simulink model "Demo_CooperativeDriving_cs"  (R2014b)
settings: Solver=ode5  SolverMode=SingleTasking  StartTime=0.0  StopTime=8  FixedStep=1/20  RelTol=1e-3
PreLoadFcn:
  | mbxruntime.callbacks.PreLoadFcn(bdroot);
  | check_NUTS_defined
  | model_closed = 0;
  | assignin('base',['model_closed_' bdroot],false);
PostLoadFcn:
  | mbxruntime.callbacks.PostLoadFcn(bdroot);
InitFcn:
  | mbxruntime.callbacks.InitFcn(bdroot);
StartFcn:
  | mbxruntime.callbacks.StartFcn(bdroot);
StopFcn:
  | mbxruntime.callbacks.StopFcn(bdroot);;
  | 
model workspace: external: MAT-File .\Demo_CooperativeDriving_cs_hws.mat (data not in the file)
undefined symbols (not defined in the file or in its folder): Cf, Cr, Jzz, Kaa, Kf, Kr, Kva, laa, lva, m, Mu, relax_on, sigma_f, sigma_r, TyreType
undefined symbols (not defined in the file): Demo_CooperativeDriving_cs_019e31e1e3c8ec68, Demo_CooperativeDriving_cs_06ab175f8e490aca, Demo_CooperativeDriving_cs_0e8790fd2fe2c963, Demo_CooperativeDriving_cs_18427a499ef3a070, Demo_CooperativeDriving_cs_19ee9ca2bc3a81c5, Demo_CooperativeDriving_cs_1e89904560c1227b, Demo_CooperativeDriving_cs_2a21be70e9dcad5a, Demo_CooperativeDriving_cs_3c5a74ebc1eb48ac, Demo_CooperativeDriving_cs_3ecaa3121594636b, Demo_CooperativeDriving_cs_43d52ce951fced72, Demo_CooperativeDriving_cs_475d8ea73085ad3a, Demo_CooperativeDriving_cs_4c403bcd11f4ac48, Demo_CooperativeDriving_cs_500af6239feadecf, Demo_CooperativeDriving_cs_53c9d62e9dff8a3d, Demo_CooperativeDriving_cs_63d3785fefec7df9, Demo_CooperativeDriving_cs_65798d17832a6887, Demo_CooperativeDriving_cs_684f3b729e0e35ac, Demo_CooperativeDriving_cs_7b7020bcdeec0410, Demo_CooperativeDriving_cs_803ec305ff24ac25, Demo_CooperativeDriving_cs_91ed94aee88cd921, Demo_CooperativeDriving_cs_9556f9105729d50c, Demo_CooperativeDriving_cs_9c65d481a76c7229, Demo_CooperativeDriving_cs_a1df81188d2866f5, Demo_CooperativeDriving_cs_a568973dc598679c, Demo_CooperativeDriving_cs_a8d1daa2431509ff, Demo_CooperativeDriving_cs_b3151f9b5b26be37, Demo_CooperativeDriving_cs_b4ba40b0a5f80027, Demo_CooperativeDriving_cs_c063d1b03f7840be, Demo_CooperativeDriving_cs_d5243d3d2f20e205, Demo_CooperativeDriving_cs_e247c6181801d737, Demo_CooperativeDriving_cs_fb1b7b87fe1ec171, Demo_CooperativeDriving_cs_Mazda_RX8_1_Path_pathUniqueID
libraries: PreScanSimulinkLibrary x10, simulink_extras x5
(part 5 of 5)

== system Demo_CooperativeDriving_cs/Toyota_Previa_1/SELF_Demux/compas converter/cart2compas ==
  Angle [deg] : Inport
  Constant : Constant  Value=90
  Constant1 : Constant  Value=360
  Gain : Gain  Gain=1/360
  Gain1 : Gain  Gain=360
  Gain2 : Gain  Gain=-1
  Rounding Function : Rounding
  Sum : Sum  Inputs=|-+
  Sum1 : Sum  Inputs=-+|
  Sum2 : Sum  Inputs=++|
  heading [deg] : Outport
  wires:
  Gain/1 -> Rounding Function/1
  Rounding Function/1 -> Gain1/1
  Gain1/1 -> Sum/1
  Angle [deg]/1 -> Sum1/2
  Sum/1 -> Gain2/1
  Sum1/1 -> Gain/1, Sum/2
  Constant/1 -> Sum1/1
  Gain2/1 -> Sum2/2
  Constant1/1 -> Sum2/1
  Sum2/1 -> heading [deg]/1

== system Demo_CooperativeDriving_cs/Toyota_Previa_1/Swarm Behavior/Vehicle/eq_of_motion ==
  Vx : Inport
  F_lat : Inport  Port=2
  Mz : Inport  Port=3
  Fcn1 : Fcn  Expr=u(1)*u(3)
  Gain : Gain  Gain=1/m  SaturateOnIntegerOverflow=on  OutDataTypeStr=Inherit: Same as input  ParamDataTypeStr=Inherit: Same as input
  Gain1 : Gain  Gain=1/Jzz  SaturateOnIntegerOverflow=on  OutDataTypeStr=Inherit: Same as input  ParamDataTypeStr=Inherit: Same as input
  Integrator1 : Integrator
  Integrator4 : Integrator
  Integrator5 : Integrator
  Psip : Integrator
  Sum1 : Sum  Inputs=-+  SaturateOnIntegerOverflow=on  InputSameDT=on  OutDataTypeStr=Inherit: Same as first input
  Vx0 : Fcn  Expr=u(1)*cos(u(3)) - u(2)*sin(u(3))
  "Vy " : Integrator
  Vy0 : Fcn  Expr=u(1)*sin(u(3)) + u(2)*cos(u(3))
  X3 : Mux  Inputs=3
  Xp : Mux  Inputs=3
  Xp1 : Mux  Inputs=2
  Xp2 : Mux  Inputs=3
  x_y_psi : Outport  InitialOutput=0
  dx_dy_dpsi : Outport  Port=2  InitialOutput=0
  ddy_ddpsi : Outport  Port=3  InitialOutput=0
  wires:
  Integrator1/1 -> X3/3, Xp2/3  "psi"
  X3/1 -> x_y_psi/1
  Integrator4/1 -> X3/1  "x"
  Integrator5/1 -> X3/2  "y"
  Vy0/1 -> Integrator5/1
  Vx0/1 -> Integrator4/1
  Xp2/1 -> Vy0/1, Vx0/1
  Mz/1 -> Gain1/1
  Xp1/1 -> ddy_ddpsi/1
  F_lat/1 -> Gain/1
  Sum1/1 -> Xp1/1, "Vy "/1  "dd_y"
  Fcn1/1 -> Sum1/1
  Xp/1 -> dx_dy_dpsi/1, Fcn1/1
  Gain1/1 -> Xp1/2, Psip/1  "dd_psi"
  Vx/1 -> Xp2/1, Xp/1
  Gain/1 -> Sum1/2
  "Vy "/1 -> Xp2/2, Xp/2  "d_y"
  Psip/1 -> Integrator1/1, Xp/3  "d_psi"

== system Demo_CooperativeDriving_cs/Toyota_Previa_1/Swarm Behavior/Vehicle/slip_angles ==
  note: relax_on
      | ON: 1
      | OFF: 0
  dx_dy_dpsi : Inport
  delta : Inport  Port=2
  Constant : Constant  Value=relax_on
  Constant1 : Constant  Value=relax_on
  Mux2 : Mux  Inputs=2
  Sum : Sum  Inputs=++|  SaturateOnIntegerOverflow=on  InputSameDT=on  OutDataTypeStr=Inherit: Same as first input
  Switch : Switch  Threshold=0.5  SaturateOnIntegerOverflow=on  InputSameDT=on
  Switch1 : Switch  Threshold=0.5  SaturateOnIntegerOverflow=on  InputSameDT=on
  alpha_front : Fcn  Expr=-atan( (u(2)+u(3)*lva)/u(1) )
  alpha_rear : Fcn  Expr=-atan( (u(2)-u(3)*laa)/u(1) )
  relaxation_length_front : Subsystem
  relaxation_length_rear : Subsystem
  alpha : Outport
  wires:
  Constant/1 -> Switch/2
  Constant1/1 -> Switch1/2
  Switch1/1 -> Mux2/2  "alpha_r"
  Switch/1 -> Mux2/1  "alpha_f"
  relaxation_length_rear/1(alpha_relax) -> Switch1/1
  relaxation_length_front/1(alpha_relax) -> Switch/1
  alpha_rear/1 -> Switch1/3, relaxation_length_rear/1(alpha_stat)  "alpha_stat_r"
  Sum/1 -> Switch/3, relaxation_length_front/1(alpha_stat)  "alpha_stat_f"
  Mux2/1 -> alpha/1
  dx_dy_dpsi/1 -> relaxation_length_rear/2(dx,dy,dphi), alpha_rear/1, relaxation_length_front/2(dx,dy,dphi), alpha_front/1
  delta/1 -> Sum/1
  alpha_front/1 -> Sum/2

== system Demo_CooperativeDriving_cs/Toyota_Previa_1/Swarm Behavior/Vehicle/tyre_forces ==
  alpha : Inport
  delta : Inport  Port=2
  Demux1 : Demux  Outputs=2
  Fy : Fcn  Expr=u(2)*cos(u(1)) + u(3)
  M2 : Fcn  Expr=u(2)*lva*cos(u(1)) - u(3)*laa
  Mux : Mux  Inputs=2
  Mux2 : Mux  Inputs=3
  tyre_front : Subsystem
  tyre_rear : Subsystem
  Fy_wheels : Outport  InitialOutput=0
  F_lat : Outport  Port=2  InitialOutput=0
  Mz : Outport  Port=3  InitialOutput=0
  wires:
  delta/1 -> Mux2/1
  tyre_rear/1(Fy_r) -> Mux/2, Mux2/3  "Fy_r"
  tyre_front/1(Fy_f) -> Mux/1, Mux2/2  "Fy_f"
  Demux1/2 -> tyre_rear/1(alpha)
  Demux1/1 -> tyre_front/1(alpha)
  alpha/1 -> Demux1/1
  Mux2/1 -> Fy/1, M2/1
  Fy/1 -> F_lat/1
  M2/1 -> Mz/1
  Mux/1 -> Fy_wheels/1

== system Demo_CooperativeDriving_cs/Toyota_Yaris_1/SELF_Demux/compas converter/cart2compas ==
  Angle [deg] : Inport
  Constant : Constant  Value=90
  Constant1 : Constant  Value=360
  Gain : Gain  Gain=1/360
  Gain1 : Gain  Gain=360
  Gain2 : Gain  Gain=-1
  Rounding Function : Rounding
  Sum : Sum  Inputs=|-+
  Sum1 : Sum  Inputs=-+|
  Sum2 : Sum  Inputs=++|
  heading [deg] : Outport
  wires:
  Gain/1 -> Rounding Function/1
  Rounding Function/1 -> Gain1/1
  Gain1/1 -> Sum/1
  Angle [deg]/1 -> Sum1/2
  Sum/1 -> Gain2/1
  Sum1/1 -> Gain/1, Sum/2
  Constant/1 -> Sum1/1
  Gain2/1 -> Sum2/2
  Constant1/1 -> Sum2/1
  Sum2/1 -> heading [deg]/1

== system Demo_CooperativeDriving_cs/Toyota_Yaris_1/Swarm Behavior/Vehicle Dynamics/eq_of_motion ==
  Vx : Inport
  F_lat : Inport  Port=2
  Mz : Inport  Port=3
  Fcn1 : Fcn  Expr=u(1)*u(3)
  Gain : Gain  Gain=1/m  SaturateOnIntegerOverflow=on  OutDataTypeStr=Inherit: Same as input  ParamDataTypeStr=Inherit: Same as input
  Gain1 : Gain  Gain=1/Jzz  SaturateOnIntegerOverflow=on  OutDataTypeStr=Inherit: Same as input  ParamDataTypeStr=Inherit: Same as input
  Integrator1 : Integrator
  Integrator4 : Integrator
  Integrator5 : Integrator
  Psip : Integrator
  Sum1 : Sum  Inputs=-+  SaturateOnIntegerOverflow=on  InputSameDT=on  OutDataTypeStr=Inherit: Same as first input
  Vx0 : Fcn  Expr=u(1)*cos(u(3)) - u(2)*sin(u(3))
  "Vy " : Integrator
  Vy0 : Fcn  Expr=u(1)*sin(u(3)) + u(2)*cos(u(3))
  X3 : Mux  Inputs=3
  Xp : Mux  Inputs=3
  Xp1 : Mux  Inputs=2
  Xp2 : Mux  Inputs=3
  x_y_psi : Outport  InitialOutput=0
  dx_dy_dpsi : Outport  Port=2  InitialOutput=0
  ddy_ddpsi : Outport  Port=3  InitialOutput=0
  wires:
  Integrator1/1 -> X3/3, Xp2/3  "psi"
  X3/1 -> x_y_psi/1
  Integrator4/1 -> X3/1  "x"
  Integrator5/1 -> X3/2  "y"
  Vy0/1 -> Integrator5/1
  Vx0/1 -> Integrator4/1
  Xp2/1 -> Vy0/1, Vx0/1
  Mz/1 -> Gain1/1
  Xp1/1 -> ddy_ddpsi/1
  F_lat/1 -> Gain/1
  Sum1/1 -> Xp1/1, "Vy "/1  "dd_y"
  Fcn1/1 -> Sum1/1
  Xp/1 -> dx_dy_dpsi/1, Fcn1/1
  Gain1/1 -> Xp1/2, Psip/1  "dd_psi"
  Vx/1 -> Xp2/1, Xp/1
  Gain/1 -> Sum1/2
  "Vy "/1 -> Xp2/2, Xp/2  "d_y"
  Psip/1 -> Integrator1/1, Xp/3  "d_psi"

== system Demo_CooperativeDriving_cs/Toyota_Yaris_1/Swarm Behavior/Vehicle Dynamics/slip_angles ==
  note: relax_on
      | ON: 1
      | OFF: 0
  dx_dy_dpsi : Inport
  delta : Inport  Port=2
  Constant : Constant  Value=relax_on
  Constant1 : Constant  Value=relax_on
  Mux2 : Mux  Inputs=2
  Sum : Sum  Inputs=++|  SaturateOnIntegerOverflow=on  InputSameDT=on  OutDataTypeStr=Inherit: Same as first input
  Switch : Switch  Threshold=0.5  SaturateOnIntegerOverflow=on  InputSameDT=on
  Switch1 : Switch  Threshold=0.5  SaturateOnIntegerOverflow=on  InputSameDT=on
  alpha_front : Fcn  Expr=-atan( (u(2)+u(3)*lva)/u(1) )
  alpha_rear : Fcn  Expr=-atan( (u(2)-u(3)*laa)/u(1) )
  relaxation_length_front : Subsystem
  relaxation_length_rear : Subsystem
  alpha : Outport
  wires:
  Constant/1 -> Switch/2
  Constant1/1 -> Switch1/2
  Switch1/1 -> Mux2/2  "alpha_r"
  Switch/1 -> Mux2/1  "alpha_f"
  relaxation_length_rear/1(alpha_relax) -> Switch1/1
  relaxation_length_front/1(alpha_relax) -> Switch/1
  alpha_rear/1 -> Switch1/3, relaxation_length_rear/1(alpha_stat)  "alpha_stat_r"
  Sum/1 -> Switch/3, relaxation_length_front/1(alpha_stat)  "alpha_stat_f"
  Mux2/1 -> alpha/1
  dx_dy_dpsi/1 -> relaxation_length_rear/2(dx,dy,dphi), alpha_rear/1, relaxation_length_front/2(dx,dy,dphi), alpha_front/1
  delta/1 -> Sum/1
  alpha_front/1 -> Sum/2

== system Demo_CooperativeDriving_cs/Toyota_Yaris_1/Swarm Behavior/Vehicle Dynamics/tyre_forces ==
  alpha : Inport
  delta : Inport  Port=2
  Demux1 : Demux  Outputs=2
  Fy : Fcn  Expr=u(2)*cos(u(1)) + u(3)
  M2 : Fcn  Expr=u(2)*lva*cos(u(1)) - u(3)*laa
  Mux : Mux  Inputs=2
  Mux2 : Mux  Inputs=3
  tyre_front : Subsystem
  tyre_rear : Subsystem
  Fy_wheels : Outport  InitialOutput=0
  F_lat : Outport  Port=2  InitialOutput=0
  Mz : Outport  Port=3  InitialOutput=0
  wires:
  delta/1 -> Mux2/1
  tyre_rear/1(Fy_r) -> Mux/2, Mux2/3  "Fy_r"
  tyre_front/1(Fy_f) -> Mux/1, Mux2/2  "Fy_f"
  Demux1/2 -> tyre_rear/1(alpha)
  Demux1/1 -> tyre_front/1(alpha)
  alpha/1 -> Demux1/1
  Mux2/1 -> Fy/1, M2/1
  Fy/1 -> F_lat/1
  M2/1 -> Mz/1
  Mux/1 -> Fy_wheels/1

== system Demo_CooperativeDriving_cs/BMW_X5_1/Swarm Behavior/Vehicle Dynamics/slip_angles/relaxation_length_front ==
  alpha_stat : Inport
  dx,dy,dphi : Inport  Port=2
  Integrator : Integrator
  Linl : Fcn  Expr=(u(4) - u(5))/(sigma_f/u(1))
  Mux2 : Mux  Inputs={3,1,1}
  alpha_relax : Outport
  wires:
  alpha_stat/1 -> Mux2/2
  dx,dy,dphi/1 -> Mux2/1
  Integrator/1 -> Mux2/3, alpha_relax/1
  Linl/1 -> Integrator/1
  Mux2/1 -> Linl/1

== system Demo_CooperativeDriving_cs/BMW_X5_1/Swarm Behavior/Vehicle Dynamics/slip_angles/relaxation_length_rear ==
  alpha_stat : Inport
  dx,dy,dphi : Inport  Port=2
  Integrator : Integrator
  Linl : Fcn  Expr=(u(4) - u(5))/(sigma_r/u(1))
  Mux2 : Mux  Inputs={3,1,1}
  alpha_relax : Outport
  wires:
  alpha_stat/1 -> Mux2/2
  dx,dy,dphi/1 -> Mux2/1
  Integrator/1 -> Mux2/3, alpha_relax/1
  Linl/1 -> Integrator/1
  Mux2/1 -> Linl/1

== system Demo_CooperativeDriving_cs/BMW_X5_1/Swarm Behavior/Vehicle Dynamics/tyre_forces/tyre_front ==
  alpha : Inport
  Borstel : Subsystem
  Exponent : Subsystem
  Fva : Fcn  Expr=Kva*u
  Fz : Constant  Value=2*Cf
  Kf : Constant  Value=Kf
  Mu : Constant  Value=Mu
  Multiport Switch : MultiPortSwitch  SaturateOnIntegerOverflow=on  InputSameDT=on
  Type : Constant  Value=TyreType
  Fy_f : Outport  InitialOutput=0
  wires:
  Fz/1 -> Exponent/2(Fz), Borstel/2(Fz)
  Mu/1 -> Exponent/3(Mu), Borstel/3(Mu)
  alpha/1 -> Fva/1, Exponent/1(alpha), Borstel/1(alpha)
  Kf/1 -> Exponent/4(Kt), Borstel/4(Kt)
  Borstel/1(Fy) -> Multiport Switch/4
  Exponent/1(Fy) -> Multiport Switch/3
  Fva/1 -> Multiport Switch/2
  Multiport Switch/1 -> Fy_f/1
  Type/1 -> Multiport Switch/1

== system Demo_CooperativeDriving_cs/BMW_X5_1/Swarm Behavior/Vehicle Dynamics/tyre_forces/tyre_rear ==
  alpha : Inport
  Borstel : Subsystem
  Exponent : Subsystem
  Fva : Fcn  Expr=Kaa*u
  Fz : Constant  Value=2*Cr
  Kr : Constant  Value=Kr
  Mu : Constant  Value=Mu
  Multiport Switch : MultiPortSwitch  SaturateOnIntegerOverflow=on  InputSameDT=on
  Type : Constant  Value=TyreType
  Fy_r : Outport  InitialOutput=0
  wires:
  alpha/1 -> Fva/1, Exponent/1(alpha), Borstel/1(alpha)
  Fz/1 -> Exponent/2(Fz), Borstel/2(Fz)
  Mu/1 -> Exponent/3(Mu), Borstel/3(Mu)
  Kr/1 -> Exponent/4(Kt), Borstel/4(Kt)
  Borstel/1(Fy) -> Multiport Switch/4
  Exponent/1(Fy) -> Multiport Switch/3
  Fva/1 -> Multiport Switch/2
  Type/1 -> Multiport Switch/1
  Multiport Switch/1 -> Fy_r/1

== system Demo_CooperativeDriving_cs/Citroen_C3_1/Swarm Behavior/Vehicle Dynamics/slip_angles/relaxation_length_front ==
  alpha_stat : Inport
  dx,dy,dphi : Inport  Port=2
  Integrator : Integrator
  Linl : Fcn  Expr=(u(4) - u(5))/(sigma_f/u(1))
  Mux2 : Mux  Inputs={3,1,1}
  alpha_relax : Outport
  wires:
  alpha_stat/1 -> Mux2/2
  dx,dy,dphi/1 -> Mux2/1
  Integrator/1 -> Mux2/3, alpha_relax/1
  Linl/1 -> Integrator/1
  Mux2/1 -> Linl/1

== system Demo_CooperativeDriving_cs/Citroen_C3_1/Swarm Behavior/Vehicle Dynamics/slip_angles/relaxation_length_rear ==
  alpha_stat : Inport
  dx,dy,dphi : Inport  Port=2
  Integrator : Integrator
  Linl : Fcn  Expr=(u(4) - u(5))/(sigma_r/u(1))
  Mux2 : Mux  Inputs={3,1,1}
  alpha_relax : Outport
  wires:
  alpha_stat/1 -> Mux2/2
  dx,dy,dphi/1 -> Mux2/1
  Integrator/1 -> Mux2/3, alpha_relax/1
  Linl/1 -> Integrator/1
  Mux2/1 -> Linl/1

== system Demo_CooperativeDriving_cs/Citroen_C3_1/Swarm Behavior/Vehicle Dynamics/tyre_forces/tyre_front ==
  alpha : Inport
  Borstel : Subsystem
  Exponent : Subsystem
  Fva : Fcn  Expr=Kva*u
  Fz : Constant  Value=2*Cf
  Kf : Constant  Value=Kf
  Mu : Constant  Value=Mu
  Multiport Switch : MultiPortSwitch  SaturateOnIntegerOverflow=on  InputSameDT=on
  Type : Constant  Value=TyreType
  Fy_f : Outport  InitialOutput=0
  wires:
  Fz/1 -> Exponent/2(Fz), Borstel/2(Fz)
  Mu/1 -> Exponent/3(Mu), Borstel/3(Mu)
  alpha/1 -> Fva/1, Exponent/1(alpha), Borstel/1(alpha)
  Kf/1 -> Exponent/4(Kt), Borstel/4(Kt)
  Borstel/1(Fy) -> Multiport Switch/4
  Exponent/1(Fy) -> Multiport Switch/3
  Fva/1 -> Multiport Switch/2
  Multiport Switch/1 -> Fy_f/1
  Type/1 -> Multiport Switch/1

== system Demo_CooperativeDriving_cs/Citroen_C3_1/Swarm Behavior/Vehicle Dynamics/tyre_forces/tyre_rear ==
  alpha : Inport
  Borstel : Subsystem
  Exponent : Subsystem
  Fva : Fcn  Expr=Kaa*u
  Fz : Constant  Value=2*Cr
  Kr : Constant  Value=Kr
  Mu : Constant  Value=Mu
  Multiport Switch : MultiPortSwitch  SaturateOnIntegerOverflow=on  InputSameDT=on
  Type : Constant  Value=TyreType
  Fy_r : Outport  InitialOutput=0
  wires:
  alpha/1 -> Fva/1, Exponent/1(alpha), Borstel/1(alpha)
  Fz/1 -> Exponent/2(Fz), Borstel/2(Fz)
  Mu/1 -> Exponent/3(Mu), Borstel/3(Mu)
  Kr/1 -> Exponent/4(Kt), Borstel/4(Kt)
  Borstel/1(Fy) -> Multiport Switch/4
  Exponent/1(Fy) -> Multiport Switch/3
  Fva/1 -> Multiport Switch/2
  Type/1 -> Multiport Switch/1
  Multiport Switch/1 -> Fy_r/1

== system Demo_CooperativeDriving_cs/Nissan_Cabstar_1/Swarm Behavior/Vehicle Dynamics/slip_angles/relaxation_length_front ==
  alpha_stat : Inport
  dx,dy,dphi : Inport  Port=2
  Integrator : Integrator
  Linl : Fcn  Expr=(u(4) - u(5))/(sigma_f/u(1))
  Mux2 : Mux  Inputs={3,1,1}
  alpha_relax : Outport
  wires:
  alpha_stat/1 -> Mux2/2
  dx,dy,dphi/1 -> Mux2/1
  Integrator/1 -> Mux2/3, alpha_relax/1
  Linl/1 -> Integrator/1
  Mux2/1 -> Linl/1

== system Demo_CooperativeDriving_cs/Nissan_Cabstar_1/Swarm Behavior/Vehicle Dynamics/slip_angles/relaxation_length_rear ==
  alpha_stat : Inport
  dx,dy,dphi : Inport  Port=2
  Integrator : Integrator
  Linl : Fcn  Expr=(u(4) - u(5))/(sigma_r/u(1))
  Mux2 : Mux  Inputs={3,1,1}
  alpha_relax : Outport
  wires:
  alpha_stat/1 -> Mux2/2
  dx,dy,dphi/1 -> Mux2/1
  Integrator/1 -> Mux2/3, alpha_relax/1
  Linl/1 -> Integrator/1
  Mux2/1 -> Linl/1

== system Demo_CooperativeDriving_cs/Nissan_Cabstar_1/Swarm Behavior/Vehicle Dynamics/tyre_forces/tyre_front ==
  alpha : Inport
  Borstel : Subsystem
  Exponent : Subsystem
  Fva : Fcn  Expr=Kva*u
  Fz : Constant  Value=2*Cf
  Kf : Constant  Value=Kf
  Mu : Constant  Value=Mu
  Multiport Switch : MultiPortSwitch  SaturateOnIntegerOverflow=on  InputSameDT=on
  Type : Constant  Value=TyreType
  Fy_f : Outport  InitialOutput=0
  wires:
  Fz/1 -> Exponent/2(Fz), Borstel/2(Fz)
  Mu/1 -> Exponent/3(Mu), Borstel/3(Mu)
  alpha/1 -> Fva/1, Exponent/1(alpha), Borstel/1(alpha)
  Kf/1 -> Exponent/4(Kt), Borstel/4(Kt)
  Borstel/1(Fy) -> Multiport Switch/4
  Exponent/1(Fy) -> Multiport Switch/3
  Fva/1 -> Multiport Switch/2
  Multiport Switch/1 -> Fy_f/1
  Type/1 -> Multiport Switch/1

== system Demo_CooperativeDriving_cs/Nissan_Cabstar_1/Swarm Behavior/Vehicle Dynamics/tyre_forces/tyre_rear ==
  alpha : Inport
  Borstel : Subsystem
  Exponent : Subsystem
  Fva : Fcn  Expr=Kaa*u
  Fz : Constant  Value=2*Cr
  Kr : Constant  Value=Kr
  Mu : Constant  Value=Mu
  Multiport Switch : MultiPortSwitch  SaturateOnIntegerOverflow=on  InputSameDT=on
  Type : Constant  Value=TyreType
  Fy_r : Outport  InitialOutput=0
  wires:
  alpha/1 -> Fva/1, Exponent/1(alpha), Borstel/1(alpha)
  Fz/1 -> Exponent/2(Fz), Borstel/2(Fz)
  Mu/1 -> Exponent/3(Mu), Borstel/3(Mu)
  Kr/1 -> Exponent/4(Kt), Borstel/4(Kt)
  Borstel/1(Fy) -> Multiport Switch/4
  Exponent/1(Fy) -> Multiport Switch/3
  Fva/1 -> Multiport Switch/2
  Type/1 -> Multiport Switch/1
  Multiport Switch/1 -> Fy_r/1

== system Demo_CooperativeDriving_cs/Toyota_Previa_1/Swarm Behavior/Vehicle/slip_angles/relaxation_length_front ==
  alpha_stat : Inport
  dx,dy,dphi : Inport  Port=2
  Integrator : Integrator
  Linl : Fcn  Expr=(u(4) - u(5))/(sigma_f/u(1))
  Mux2 : Mux  Inputs={3,1,1}
  alpha_relax : Outport
  wires:
  alpha_stat/1 -> Mux2/2
  dx,dy,dphi/1 -> Mux2/1
  Integrator/1 -> Mux2/3, alpha_relax/1
  Linl/1 -> Integrator/1
  Mux2/1 -> Linl/1

== system Demo_CooperativeDriving_cs/Toyota_Previa_1/Swarm Behavior/Vehicle/slip_angles/relaxation_length_rear ==
  alpha_stat : Inport
  dx,dy,dphi : Inport  Port=2
  Integrator : Integrator
  Linl : Fcn  Expr=(u(4) - u(5))/(sigma_r/u(1))
  Mux2 : Mux  Inputs={3,1,1}
  alpha_relax : Outport
  wires:
  alpha_stat/1 -> Mux2/2
  dx,dy,dphi/1 -> Mux2/1
  Integrator/1 -> Mux2/3, alpha_relax/1
  Linl/1 -> Integrator/1
  Mux2/1 -> Linl/1

== system Demo_CooperativeDriving_cs/Toyota_Previa_1/Swarm Behavior/Vehicle/tyre_forces/tyre_front ==
  alpha : Inport
  Borstel : Subsystem
  Exponent : Subsystem
  Fva : Fcn  Expr=Kva*u
  Fz : Constant  Value=2*Cf
  Kf : Constant  Value=Kf
  Mu : Constant  Value=Mu
  Multiport Switch : MultiPortSwitch  SaturateOnIntegerOverflow=on  InputSameDT=on
  Type : Constant  Value=TyreType
  Fy_f : Outport  InitialOutput=0
  wires:
  Fz/1 -> Exponent/2(Fz), Borstel/2(Fz)
  Mu/1 -> Exponent/3(Mu), Borstel/3(Mu)
  alpha/1 -> Fva/1, Exponent/1(alpha), Borstel/1(alpha)
  Kf/1 -> Exponent/4(Kt), Borstel/4(Kt)
  Borstel/1(Fy) -> Multiport Switch/4
  Exponent/1(Fy) -> Multiport Switch/3
  Fva/1 -> Multiport Switch/2
  Multiport Switch/1 -> Fy_f/1
  Type/1 -> Multiport Switch/1

== system Demo_CooperativeDriving_cs/Toyota_Previa_1/Swarm Behavior/Vehicle/tyre_forces/tyre_rear ==
  alpha : Inport
  Borstel : Subsystem
  Exponent : Subsystem
  Fva : Fcn  Expr=Kaa*u
  Fz : Constant  Value=2*Cr
  Kr : Constant  Value=Kr
  Mu : Constant  Value=Mu
  Multiport Switch : MultiPortSwitch  SaturateOnIntegerOverflow=on  InputSameDT=on
  Type : Constant  Value=TyreType
  Fy_r : Outport  InitialOutput=0
  wires:
  alpha/1 -> Fva/1, Exponent/1(alpha), Borstel/1(alpha)
  Fz/1 -> Exponent/2(Fz), Borstel/2(Fz)
  Mu/1 -> Exponent/3(Mu), Borstel/3(Mu)
  Kr/1 -> Exponent/4(Kt), Borstel/4(Kt)
  Borstel/1(Fy) -> Multiport Switch/4
  Exponent/1(Fy) -> Multiport Switch/3
  Fva/1 -> Multiport Switch/2
  Type/1 -> Multiport Switch/1
  Multiport Switch/1 -> Fy_r/1

== system Demo_CooperativeDriving_cs/Toyota_Yaris_1/Swarm Behavior/Vehicle Dynamics/slip_angles/relaxation_length_front ==
  alpha_stat : Inport
  dx,dy,dphi : Inport  Port=2
  Integrator : Integrator
  Linl : Fcn  Expr=(u(4) - u(5))/(sigma_f/u(1))
  Mux2 : Mux  Inputs={3,1,1}
  alpha_relax : Outport
  wires:
  alpha_stat/1 -> Mux2/2
  dx,dy,dphi/1 -> Mux2/1
  Integrator/1 -> Mux2/3, alpha_relax/1
  Linl/1 -> Integrator/1
  Mux2/1 -> Linl/1

== system Demo_CooperativeDriving_cs/Toyota_Yaris_1/Swarm Behavior/Vehicle Dynamics/slip_angles/relaxation_length_rear ==
  alpha_stat : Inport
  dx,dy,dphi : Inport  Port=2
  Integrator : Integrator
  Linl : Fcn  Expr=(u(4) - u(5))/(sigma_r/u(1))
  Mux2 : Mux  Inputs={3,1,1}
  alpha_relax : Outport
  wires:
  alpha_stat/1 -> Mux2/2
  dx,dy,dphi/1 -> Mux2/1
  Integrator/1 -> Mux2/3, alpha_relax/1
  Linl/1 -> Integrator/1
  Mux2/1 -> Linl/1

== system Demo_CooperativeDriving_cs/Toyota_Yaris_1/Swarm Behavior/Vehicle Dynamics/tyre_forces/tyre_front ==
  alpha : Inport
  Borstel : Subsystem
  Exponent : Subsystem
  Fva : Fcn  Expr=Kva*u
  Fz : Constant  Value=2*Cf
  Kf : Constant  Value=Kf
  Mu : Constant  Value=Mu
  Multiport Switch : MultiPortSwitch  SaturateOnIntegerOverflow=on  InputSameDT=on
  Type : Constant  Value=TyreType
  Fy_f : Outport  InitialOutput=0
  wires:
  Fz/1 -> Exponent/2(Fz), Borstel/2(Fz)
  Mu/1 -> Exponent/3(Mu), Borstel/3(Mu)
  alpha/1 -> Fva/1, Exponent/1(alpha), Borstel/1(alpha)
  Kf/1 -> Exponent/4(Kt), Borstel/4(Kt)
  Borstel/1(Fy) -> Multiport Switch/4
  Exponent/1(Fy) -> Multiport Switch/3
  Fva/1 -> Multiport Switch/2
  Multiport Switch/1 -> Fy_f/1
  Type/1 -> Multiport Switch/1

== system Demo_CooperativeDriving_cs/Toyota_Yaris_1/Swarm Behavior/Vehicle Dynamics/tyre_forces/tyre_rear ==
  alpha : Inport
  Borstel : Subsystem
  Exponent : Subsystem
  Fva : Fcn  Expr=Kaa*u
  Fz : Constant  Value=2*Cr
  Kr : Constant  Value=Kr
  Mu : Constant  Value=Mu
  Multiport Switch : MultiPortSwitch  SaturateOnIntegerOverflow=on  InputSameDT=on
  Type : Constant  Value=TyreType
  Fy_r : Outport  InitialOutput=0
  wires:
  alpha/1 -> Fva/1, Exponent/1(alpha), Borstel/1(alpha)
  Fz/1 -> Exponent/2(Fz), Borstel/2(Fz)
  Mu/1 -> Exponent/3(Mu), Borstel/3(Mu)
  Kr/1 -> Exponent/4(Kt), Borstel/4(Kt)
  Borstel/1(Fy) -> Multiport Switch/4
  Exponent/1(Fy) -> Multiport Switch/3
  Fva/1 -> Multiport Switch/2
  Type/1 -> Multiport Switch/1
  Multiport Switch/1 -> Fy_r/1

== system Demo_CooperativeDriving_cs/BMW_X5_1/Swarm Behavior/Vehicle Dynamics/tyre_forces/tyre_front/Borstel ==
  alpha : Inport
  Fz : Inport  Port=2
  Mu : Inport  Port=3
  Kt : Inport  Port=4
  Abs : Abs  SaturateOnIntegerOverflow=on
  F : Fcn  Expr=(3*u(2) - 3*u(2)^2 + u(2)^3)*u(1)
  Fmax : Fcn  Expr=u(1)
  Gain : Gain  Gain=1/3  SaturateOnIntegerOverflow=on  OutDataTypeStr=Inherit: Same as input  ParamDataTypeStr=Inherit: Same as input
  Math Function : Math  Operator=reciprocal  SaturateOnIntegerOverflow=on
  Mux1 : Mux  Inputs=2
  Product : Product  SaturateOnIntegerOverflow=on  RndMeth=Zero  InputSameDT=on  OutDataTypeStr=Inherit: Same as first input
  Product1 : Product  Inputs=3  SaturateOnIntegerOverflow=on  RndMeth=Zero  InputSameDT=on  OutDataTypeStr=Inherit: Same as first input
  Relational Operator : RelationalOperator  InputSameDT=on
  Sign : Signum
  Switch : Switch  Threshold=0.5  SaturateOnIntegerOverflow=on  InputSameDT=on
  Trigonometric Function : Trigonometry  Operator=tan
  Fy : Outport
  wires:
  Abs/1 -> Relational Operator/1, Product/1
  Kt/1 -> Gain/1
  Relational Operator/1 -> Switch/2
  Trigonometric Function/1 -> Abs/1
  Mux1/1 -> F/1, Fmax/1
  Sign/1 -> Mux1/1
  Product/1 -> Mux1/2
  F/1 -> Switch/3
  Fmax/1 -> Switch/1
  alpha/1 -> Trigonometric Function/1, Sign/1
  Switch/1 -> Product1/1
  Product1/1 -> Fy/1
  Fz/1 -> Product1/2
  Mu/1 -> Product1/3
  Gain/1 -> Product/2, Math Function/1
  Math Function/1 -> Relational Operator/2

== system Demo_CooperativeDriving_cs/BMW_X5_1/Swarm Behavior/Vehicle Dynamics/tyre_forces/tyre_front/Exponent ==
  alpha : Inport
  Fz : Inport  Port=2
  Mu : Inport  Port=3
  Kt : Inport  Port=4
  Abs : Abs  SaturateOnIntegerOverflow=on
  MuY Front Wheels : Fcn  Expr=(1 - exp(-u(2)*u(1)))
  Mux1 : Mux  Inputs=2
  Product : Product  Inputs=4  SaturateOnIntegerOverflow=on  RndMeth=Zero  InputSameDT=on  OutDataTypeStr=Inherit: Same as first input
  Saturation2 : Saturate  UpperLimit=inf  LowerLimit=1e-9
  Sign : Signum
  Fy : Outport
  wires:
  Abs/1 -> Saturation2/1
  Saturation2/1 -> Mux1/1
  Mux1/1 -> MuY Front Wheels/1
  Kt/1 -> Mux1/2
  Sign/1 -> Product/1
  MuY Front Wheels/1 -> Product/2
  alpha/1 -> Abs/1, Sign/1
  Product/1 -> Fy/1
  Fz/1 -> Product/3
  Mu/1 -> Product/4

== system Demo_CooperativeDriving_cs/BMW_X5_1/Swarm Behavior/Vehicle Dynamics/tyre_forces/tyre_rear/Borstel ==
  alpha : Inport
  Fz : Inport  Port=2
  Mu : Inport  Port=3
  Kt : Inport  Port=4
  Abs : Abs  SaturateOnIntegerOverflow=on
  F : Fcn  Expr=(3*u(2) - 3*u(2)^2 + u(2)^3)*u(1)
  Fmax : Fcn  Expr=u(1)
  Gain : Gain  Gain=1/3  SaturateOnIntegerOverflow=on  OutDataTypeStr=Inherit: Same as input  ParamDataTypeStr=Inherit: Same as input
  Math Function : Math  Operator=reciprocal  SaturateOnIntegerOverflow=on
  Mux1 : Mux  Inputs=2
  Product : Product  SaturateOnIntegerOverflow=on  RndMeth=Zero  InputSameDT=on  OutDataTypeStr=Inherit: Same as first input
  Product1 : Product  Inputs=3  SaturateOnIntegerOverflow=on  RndMeth=Zero  InputSameDT=on  OutDataTypeStr=Inherit: Same as first input
  Relational Operator : RelationalOperator  InputSameDT=on
  Sign : Signum
  Switch : Switch  Threshold=0.5  SaturateOnIntegerOverflow=on  InputSameDT=on
  Trigonometric Function : Trigonometry  Operator=tan
  Fy : Outport
  wires:
  Abs/1 -> Relational Operator/1, Product/1
  Kt/1 -> Gain/1
  Relational Operator/1 -> Switch/2
  Trigonometric Function/1 -> Abs/1
  Mux1/1 -> F/1, Fmax/1
  Sign/1 -> Mux1/1
  Product/1 -> Mux1/2
  F/1 -> Switch/3
  Fmax/1 -> Switch/1
  alpha/1 -> Trigonometric Function/1, Sign/1
  Switch/1 -> Product1/1
  Product1/1 -> Fy/1
  Fz/1 -> Product1/2
  Mu/1 -> Product1/3
  Gain/1 -> Product/2, Math Function/1
  Math Function/1 -> Relational Operator/2

== system Demo_CooperativeDriving_cs/BMW_X5_1/Swarm Behavior/Vehicle Dynamics/tyre_forces/tyre_rear/Exponent ==
  alpha : Inport
  Fz : Inport  Port=2
  Mu : Inport  Port=3
  Kt : Inport  Port=4
  Abs : Abs  SaturateOnIntegerOverflow=on
  MuY Front Wheels : Fcn  Expr=(1 - exp(-u(2)*u(1)))
  Mux1 : Mux  Inputs=2
  Product : Product  Inputs=4  SaturateOnIntegerOverflow=on  RndMeth=Zero  InputSameDT=on  OutDataTypeStr=Inherit: Same as first input
  Saturation2 : Saturate  UpperLimit=inf  LowerLimit=1e-9
  Sign : Signum
  Fy : Outport
  wires:
  Abs/1 -> Saturation2/1
  Saturation2/1 -> Mux1/1
  Mux1/1 -> MuY Front Wheels/1
  Kt/1 -> Mux1/2
  Sign/1 -> Product/1
  MuY Front Wheels/1 -> Product/2
  alpha/1 -> Abs/1, Sign/1
  Product/1 -> Fy/1
  Fz/1 -> Product/3
  Mu/1 -> Product/4

== system Demo_CooperativeDriving_cs/Citroen_C3_1/Swarm Behavior/Vehicle Dynamics/tyre_forces/tyre_front/Borstel ==
  alpha : Inport
  Fz : Inport  Port=2
  Mu : Inport  Port=3
  Kt : Inport  Port=4
  Abs : Abs  SaturateOnIntegerOverflow=on
  F : Fcn  Expr=(3*u(2) - 3*u(2)^2 + u(2)^3)*u(1)
  Fmax : Fcn  Expr=u(1)
  Gain : Gain  Gain=1/3  SaturateOnIntegerOverflow=on  OutDataTypeStr=Inherit: Same as input  ParamDataTypeStr=Inherit: Same as input
  Math Function : Math  Operator=reciprocal  SaturateOnIntegerOverflow=on
  Mux1 : Mux  Inputs=2
  Product : Product  SaturateOnIntegerOverflow=on  RndMeth=Zero  InputSameDT=on  OutDataTypeStr=Inherit: Same as first input
  Product1 : Product  Inputs=3  SaturateOnIntegerOverflow=on  RndMeth=Zero  InputSameDT=on  OutDataTypeStr=Inherit: Same as first input
  Relational Operator : RelationalOperator  InputSameDT=on
  Sign : Signum
  Switch : Switch  Threshold=0.5  SaturateOnIntegerOverflow=on  InputSameDT=on
  Trigonometric Function : Trigonometry  Operator=tan
  Fy : Outport
  wires:
  Abs/1 -> Relational Operator/1, Product/1
  Kt/1 -> Gain/1
  Relational Operator/1 -> Switch/2
  Trigonometric Function/1 -> Abs/1
  Mux1/1 -> F/1, Fmax/1
  Sign/1 -> Mux1/1
  Product/1 -> Mux1/2
  F/1 -> Switch/3
  Fmax/1 -> Switch/1
  alpha/1 -> Trigonometric Function/1, Sign/1
  Switch/1 -> Product1/1
  Product1/1 -> Fy/1
  Fz/1 -> Product1/2
  Mu/1 -> Product1/3
  Gain/1 -> Product/2, Math Function/1
  Math Function/1 -> Relational Operator/2

== system Demo_CooperativeDriving_cs/Citroen_C3_1/Swarm Behavior/Vehicle Dynamics/tyre_forces/tyre_front/Exponent ==
  alpha : Inport
  Fz : Inport  Port=2
  Mu : Inport  Port=3
  Kt : Inport  Port=4
  Abs : Abs  SaturateOnIntegerOverflow=on
  MuY Front Wheels : Fcn  Expr=(1 - exp(-u(2)*u(1)))
  Mux1 : Mux  Inputs=2
  Product : Product  Inputs=4  SaturateOnIntegerOverflow=on  RndMeth=Zero  InputSameDT=on  OutDataTypeStr=Inherit: Same as first input
  Saturation2 : Saturate  UpperLimit=inf  LowerLimit=1e-9
  Sign : Signum
  Fy : Outport
  wires:
  Abs/1 -> Saturation2/1
  Saturation2/1 -> Mux1/1
  Mux1/1 -> MuY Front Wheels/1
  Kt/1 -> Mux1/2
  Sign/1 -> Product/1
  MuY Front Wheels/1 -> Product/2
  alpha/1 -> Abs/1, Sign/1
  Product/1 -> Fy/1
  Fz/1 -> Product/3
  Mu/1 -> Product/4

== system Demo_CooperativeDriving_cs/Citroen_C3_1/Swarm Behavior/Vehicle Dynamics/tyre_forces/tyre_rear/Borstel ==
  alpha : Inport
  Fz : Inport  Port=2
  Mu : Inport  Port=3
  Kt : Inport  Port=4
  Abs : Abs  SaturateOnIntegerOverflow=on
  F : Fcn  Expr=(3*u(2) - 3*u(2)^2 + u(2)^3)*u(1)
  Fmax : Fcn  Expr=u(1)
  Gain : Gain  Gain=1/3  SaturateOnIntegerOverflow=on  OutDataTypeStr=Inherit: Same as input  ParamDataTypeStr=Inherit: Same as input
  Math Function : Math  Operator=reciprocal  SaturateOnIntegerOverflow=on
  Mux1 : Mux  Inputs=2
  Product : Product  SaturateOnIntegerOverflow=on  RndMeth=Zero  InputSameDT=on  OutDataTypeStr=Inherit: Same as first input
  Product1 : Product  Inputs=3  SaturateOnIntegerOverflow=on  RndMeth=Zero  InputSameDT=on  OutDataTypeStr=Inherit: Same as first input
  Relational Operator : RelationalOperator  InputSameDT=on
  Sign : Signum
  Switch : Switch  Threshold=0.5  SaturateOnIntegerOverflow=on  InputSameDT=on
  Trigonometric Function : Trigonometry  Operator=tan
  Fy : Outport
  wires:
  Abs/1 -> Relational Operator/1, Product/1
  Kt/1 -> Gain/1
  Relational Operator/1 -> Switch/2
  Trigonometric Function/1 -> Abs/1
  Mux1/1 -> F/1, Fmax/1
  Sign/1 -> Mux1/1
  Product/1 -> Mux1/2
  F/1 -> Switch/3
  Fmax/1 -> Switch/1
  alpha/1 -> Trigonometric Function/1, Sign/1
  Switch/1 -> Product1/1
  Product1/1 -> Fy/1
  Fz/1 -> Product1/2
  Mu/1 -> Product1/3
  Gain/1 -> Product/2, Math Function/1
  Math Function/1 -> Relational Operator/2

== system Demo_CooperativeDriving_cs/Citroen_C3_1/Swarm Behavior/Vehicle Dynamics/tyre_forces/tyre_rear/Exponent ==
  alpha : Inport
  Fz : Inport  Port=2
  Mu : Inport  Port=3
  Kt : Inport  Port=4
  Abs : Abs  SaturateOnIntegerOverflow=on
  MuY Front Wheels : Fcn  Expr=(1 - exp(-u(2)*u(1)))
  Mux1 : Mux  Inputs=2
  Product : Product  Inputs=4  SaturateOnIntegerOverflow=on  RndMeth=Zero  InputSameDT=on  OutDataTypeStr=Inherit: Same as first input
  Saturation2 : Saturate  UpperLimit=inf  LowerLimit=1e-9
  Sign : Signum
  Fy : Outport
  wires:
  Abs/1 -> Saturation2/1
  Saturation2/1 -> Mux1/1
  Mux1/1 -> MuY Front Wheels/1
  Kt/1 -> Mux1/2
  Sign/1 -> Product/1
  MuY Front Wheels/1 -> Product/2
  alpha/1 -> Abs/1, Sign/1
  Product/1 -> Fy/1
  Fz/1 -> Product/3
  Mu/1 -> Product/4

== system Demo_CooperativeDriving_cs/Nissan_Cabstar_1/Swarm Behavior/Vehicle Dynamics/tyre_forces/tyre_front/Borstel ==
  alpha : Inport
  Fz : Inport  Port=2
  Mu : Inport  Port=3
  Kt : Inport  Port=4
  Abs : Abs  SaturateOnIntegerOverflow=on
  F : Fcn  Expr=(3*u(2) - 3*u(2)^2 + u(2)^3)*u(1)
  Fmax : Fcn  Expr=u(1)
  Gain : Gain  Gain=1/3  SaturateOnIntegerOverflow=on  OutDataTypeStr=Inherit: Same as input  ParamDataTypeStr=Inherit: Same as input
  Math Function : Math  Operator=reciprocal  SaturateOnIntegerOverflow=on
  Mux1 : Mux  Inputs=2
  Product : Product  SaturateOnIntegerOverflow=on  RndMeth=Zero  InputSameDT=on  OutDataTypeStr=Inherit: Same as first input
  Product1 : Product  Inputs=3  SaturateOnIntegerOverflow=on  RndMeth=Zero  InputSameDT=on  OutDataTypeStr=Inherit: Same as first input
  Relational Operator : RelationalOperator  InputSameDT=on
  Sign : Signum
  Switch : Switch  Threshold=0.5  SaturateOnIntegerOverflow=on  InputSameDT=on
  Trigonometric Function : Trigonometry  Operator=tan
  Fy : Outport
  wires:
  Abs/1 -> Relational Operator/1, Product/1
  Kt/1 -> Gain/1
  Relational Operator/1 -> Switch/2
  Trigonometric Function/1 -> Abs/1
  Mux1/1 -> F/1, Fmax/1
  Sign/1 -> Mux1/1
  Product/1 -> Mux1/2
  F/1 -> Switch/3
  Fmax/1 -> Switch/1
  alpha/1 -> Trigonometric Function/1, Sign/1
  Switch/1 -> Product1/1
  Product1/1 -> Fy/1
  Fz/1 -> Product1/2
  Mu/1 -> Product1/3
  Gain/1 -> Product/2, Math Function/1
  Math Function/1 -> Relational Operator/2

== system Demo_CooperativeDriving_cs/Nissan_Cabstar_1/Swarm Behavior/Vehicle Dynamics/tyre_forces/tyre_front/Exponent ==
  alpha : Inport
  Fz : Inport  Port=2
  Mu : Inport  Port=3
  Kt : Inport  Port=4
  Abs : Abs  SaturateOnIntegerOverflow=on
  MuY Front Wheels : Fcn  Expr=(1 - exp(-u(2)*u(1)))
  Mux1 : Mux  Inputs=2
  Product : Product  Inputs=4  SaturateOnIntegerOverflow=on  RndMeth=Zero  InputSameDT=on  OutDataTypeStr=Inherit: Same as first input
  Saturation2 : Saturate  UpperLimit=inf  LowerLimit=1e-9
  Sign : Signum
  Fy : Outport
  wires:
  Abs/1 -> Saturation2/1
  Saturation2/1 -> Mux1/1
  Mux1/1 -> MuY Front Wheels/1
  Kt/1 -> Mux1/2
  Sign/1 -> Product/1
  MuY Front Wheels/1 -> Product/2
  alpha/1 -> Abs/1, Sign/1
  Product/1 -> Fy/1
  Fz/1 -> Product/3
  Mu/1 -> Product/4

== system Demo_CooperativeDriving_cs/Nissan_Cabstar_1/Swarm Behavior/Vehicle Dynamics/tyre_forces/tyre_rear/Borstel ==
  alpha : Inport
  Fz : Inport  Port=2
  Mu : Inport  Port=3
  Kt : Inport  Port=4
  Abs : Abs  SaturateOnIntegerOverflow=on
  F : Fcn  Expr=(3*u(2) - 3*u(2)^2 + u(2)^3)*u(1)
  Fmax : Fcn  Expr=u(1)
  Gain : Gain  Gain=1/3  SaturateOnIntegerOverflow=on  OutDataTypeStr=Inherit: Same as input  ParamDataTypeStr=Inherit: Same as input
  Math Function : Math  Operator=reciprocal  SaturateOnIntegerOverflow=on
  Mux1 : Mux  Inputs=2
  Product : Product  SaturateOnIntegerOverflow=on  RndMeth=Zero  InputSameDT=on  OutDataTypeStr=Inherit: Same as first input
  Product1 : Product  Inputs=3  SaturateOnIntegerOverflow=on  RndMeth=Zero  InputSameDT=on  OutDataTypeStr=Inherit: Same as first input
  Relational Operator : RelationalOperator  InputSameDT=on
  Sign : Signum
  Switch : Switch  Threshold=0.5  SaturateOnIntegerOverflow=on  InputSameDT=on
  Trigonometric Function : Trigonometry  Operator=tan
  Fy : Outport
  wires:
  Abs/1 -> Relational Operator/1, Product/1
  Kt/1 -> Gain/1
  Relational Operator/1 -> Switch/2
  Trigonometric Function/1 -> Abs/1
  Mux1/1 -> F/1, Fmax/1
  Sign/1 -> Mux1/1
  Product/1 -> Mux1/2
  F/1 -> Switch/3
  Fmax/1 -> Switch/1
  alpha/1 -> Trigonometric Function/1, Sign/1
  Switch/1 -> Product1/1
  Product1/1 -> Fy/1
  Fz/1 -> Product1/2
  Mu/1 -> Product1/3
  Gain/1 -> Product/2, Math Function/1
  Math Function/1 -> Relational Operator/2

== system Demo_CooperativeDriving_cs/Nissan_Cabstar_1/Swarm Behavior/Vehicle Dynamics/tyre_forces/tyre_rear/Exponent ==
  alpha : Inport
  Fz : Inport  Port=2
  Mu : Inport  Port=3
  Kt : Inport  Port=4
  Abs : Abs  SaturateOnIntegerOverflow=on
  MuY Front Wheels : Fcn  Expr=(1 - exp(-u(2)*u(1)))
  Mux1 : Mux  Inputs=2
  Product : Product  Inputs=4  SaturateOnIntegerOverflow=on  RndMeth=Zero  InputSameDT=on  OutDataTypeStr=Inherit: Same as first input
  Saturation2 : Saturate  UpperLimit=inf  LowerLimit=1e-9
  Sign : Signum
  Fy : Outport
  wires:
  Abs/1 -> Saturation2/1
  Saturation2/1 -> Mux1/1
  Mux1/1 -> MuY Front Wheels/1
  Kt/1 -> Mux1/2
  Sign/1 -> Product/1
  MuY Front Wheels/1 -> Product/2
  alpha/1 -> Abs/1, Sign/1
  Product/1 -> Fy/1
  Fz/1 -> Product/3
  Mu/1 -> Product/4

== system Demo_CooperativeDriving_cs/Toyota_Previa_1/Swarm Behavior/Vehicle/tyre_forces/tyre_front/Borstel ==
  alpha : Inport
  Fz : Inport  Port=2
  Mu : Inport  Port=3
  Kt : Inport  Port=4
  Abs : Abs  SaturateOnIntegerOverflow=on
  F : Fcn  Expr=(3*u(2) - 3*u(2)^2 + u(2)^3)*u(1)
  Fmax : Fcn  Expr=u(1)
  Gain : Gain  Gain=1/3  SaturateOnIntegerOverflow=on  OutDataTypeStr=Inherit: Same as input  ParamDataTypeStr=Inherit: Same as input
  Math Function : Math  Operator=reciprocal  SaturateOnIntegerOverflow=on
  Mux1 : Mux  Inputs=2
  Product : Product  SaturateOnIntegerOverflow=on  RndMeth=Zero  InputSameDT=on  OutDataTypeStr=Inherit: Same as first input
  Product1 : Product  Inputs=3  SaturateOnIntegerOverflow=on  RndMeth=Zero  InputSameDT=on  OutDataTypeStr=Inherit: Same as first input
  Relational Operator : RelationalOperator  InputSameDT=on
  Sign : Signum
  Switch : Switch  Threshold=0.5  SaturateOnIntegerOverflow=on  InputSameDT=on
  Trigonometric Function : Trigonometry  Operator=tan
  Fy : Outport
  wires:
  Abs/1 -> Relational Operator/1, Product/1
  Kt/1 -> Gain/1
  Relational Operator/1 -> Switch/2
  Trigonometric Function/1 -> Abs/1
  Mux1/1 -> F/1, Fmax/1
  Sign/1 -> Mux1/1
  Product/1 -> Mux1/2
  F/1 -> Switch/3
  Fmax/1 -> Switch/1
  alpha/1 -> Trigonometric Function/1, Sign/1
  Switch/1 -> Product1/1
  Product1/1 -> Fy/1
  Fz/1 -> Product1/2
  Mu/1 -> Product1/3
  Gain/1 -> Product/2, Math Function/1
  Math Function/1 -> Relational Operator/2

== system Demo_CooperativeDriving_cs/Toyota_Previa_1/Swarm Behavior/Vehicle/tyre_forces/tyre_front/Exponent ==
  alpha : Inport
  Fz : Inport  Port=2
  Mu : Inport  Port=3
  Kt : Inport  Port=4
  Abs : Abs  SaturateOnIntegerOverflow=on
  MuY Front Wheels : Fcn  Expr=(1 - exp(-u(2)*u(1)))
  Mux1 : Mux  Inputs=2
  Product : Product  Inputs=4  SaturateOnIntegerOverflow=on  RndMeth=Zero  InputSameDT=on  OutDataTypeStr=Inherit: Same as first input
  Saturation2 : Saturate  UpperLimit=inf  LowerLimit=1e-9
  Sign : Signum
  Fy : Outport
  wires:
  Abs/1 -> Saturation2/1
  Saturation2/1 -> Mux1/1
  Mux1/1 -> MuY Front Wheels/1
  Kt/1 -> Mux1/2
  Sign/1 -> Product/1
  MuY Front Wheels/1 -> Product/2
  alpha/1 -> Abs/1, Sign/1
  Product/1 -> Fy/1
  Fz/1 -> Product/3
  Mu/1 -> Product/4

== system Demo_CooperativeDriving_cs/Toyota_Previa_1/Swarm Behavior/Vehicle/tyre_forces/tyre_rear/Borstel ==
  alpha : Inport
  Fz : Inport  Port=2
  Mu : Inport  Port=3
  Kt : Inport  Port=4
  Abs : Abs  SaturateOnIntegerOverflow=on
  F : Fcn  Expr=(3*u(2) - 3*u(2)^2 + u(2)^3)*u(1)
  Fmax : Fcn  Expr=u(1)
  Gain : Gain  Gain=1/3  SaturateOnIntegerOverflow=on  OutDataTypeStr=Inherit: Same as input  ParamDataTypeStr=Inherit: Same as input
  Math Function : Math  Operator=reciprocal  SaturateOnIntegerOverflow=on
  Mux1 : Mux  Inputs=2
  Product : Product  SaturateOnIntegerOverflow=on  RndMeth=Zero  InputSameDT=on  OutDataTypeStr=Inherit: Same as first input
  Product1 : Product  Inputs=3  SaturateOnIntegerOverflow=on  RndMeth=Zero  InputSameDT=on  OutDataTypeStr=Inherit: Same as first input
  Relational Operator : RelationalOperator  InputSameDT=on
  Sign : Signum
  Switch : Switch  Threshold=0.5  SaturateOnIntegerOverflow=on  InputSameDT=on
  Trigonometric Function : Trigonometry  Operator=tan
  Fy : Outport
  wires:
  Abs/1 -> Relational Operator/1, Product/1
  Kt/1 -> Gain/1
  Relational Operator/1 -> Switch/2
  Trigonometric Function/1 -> Abs/1
  Mux1/1 -> F/1, Fmax/1
  Sign/1 -> Mux1/1
  Product/1 -> Mux1/2
  F/1 -> Switch/3
  Fmax/1 -> Switch/1
  alpha/1 -> Trigonometric Function/1, Sign/1
  Switch/1 -> Product1/1
  Product1/1 -> Fy/1
  Fz/1 -> Product1/2
  Mu/1 -> Product1/3
  Gain/1 -> Product/2, Math Function/1
  Math Function/1 -> Relational Operator/2

== system Demo_CooperativeDriving_cs/Toyota_Previa_1/Swarm Behavior/Vehicle/tyre_forces/tyre_rear/Exponent ==
  alpha : Inport
  Fz : Inport  Port=2
  Mu : Inport  Port=3
  Kt : Inport  Port=4
  Abs : Abs  SaturateOnIntegerOverflow=on
  MuY Front Wheels : Fcn  Expr=(1 - exp(-u(2)*u(1)))
  Mux1 : Mux  Inputs=2
  Product : Product  Inputs=4  SaturateOnIntegerOverflow=on  RndMeth=Zero  InputSameDT=on  OutDataTypeStr=Inherit: Same as first input
  Saturation2 : Saturate  UpperLimit=inf  LowerLimit=1e-9
  Sign : Signum
  Fy : Outport
  wires:
  Abs/1 -> Saturation2/1
  Saturation2/1 -> Mux1/1
  Mux1/1 -> MuY Front Wheels/1
  Kt/1 -> Mux1/2
  Sign/1 -> Product/1
  MuY Front Wheels/1 -> Product/2
  alpha/1 -> Abs/1, Sign/1
  Product/1 -> Fy/1
  Fz/1 -> Product/3
  Mu/1 -> Product/4

== system Demo_CooperativeDriving_cs/Toyota_Yaris_1/Swarm Behavior/Vehicle Dynamics/tyre_forces/tyre_front/Borstel ==
  alpha : Inport
  Fz : Inport  Port=2
  Mu : Inport  Port=3
  Kt : Inport  Port=4
  Abs : Abs  SaturateOnIntegerOverflow=on
  F : Fcn  Expr=(3*u(2) - 3*u(2)^2 + u(2)^3)*u(1)
  Fmax : Fcn  Expr=u(1)
  Gain : Gain  Gain=1/3  SaturateOnIntegerOverflow=on  OutDataTypeStr=Inherit: Same as input  ParamDataTypeStr=Inherit: Same as input
  Math Function : Math  Operator=reciprocal  SaturateOnIntegerOverflow=on
  Mux1 : Mux  Inputs=2
  Product : Product  SaturateOnIntegerOverflow=on  RndMeth=Zero  InputSameDT=on  OutDataTypeStr=Inherit: Same as first input
  Product1 : Product  Inputs=3  SaturateOnIntegerOverflow=on  RndMeth=Zero  InputSameDT=on  OutDataTypeStr=Inherit: Same as first input
  Relational Operator : RelationalOperator  InputSameDT=on
  Sign : Signum
  Switch : Switch  Threshold=0.5  SaturateOnIntegerOverflow=on  InputSameDT=on
  Trigonometric Function : Trigonometry  Operator=tan
  Fy : Outport
  wires:
  Abs/1 -> Relational Operator/1, Product/1
  Kt/1 -> Gain/1
  Relational Operator/1 -> Switch/2
  Trigonometric Function/1 -> Abs/1
  Mux1/1 -> F/1, Fmax/1
  Sign/1 -> Mux1/1
  Product/1 -> Mux1/2
  F/1 -> Switch/3
  Fmax/1 -> Switch/1
  alpha/1 -> Trigonometric Function/1, Sign/1
  Switch/1 -> Product1/1
  Product1/1 -> Fy/1
  Fz/1 -> Product1/2
  Mu/1 -> Product1/3
  Gain/1 -> Product/2, Math Function/1
  Math Function/1 -> Relational Operator/2

== system Demo_CooperativeDriving_cs/Toyota_Yaris_1/Swarm Behavior/Vehicle Dynamics/tyre_forces/tyre_front/Exponent ==
  alpha : Inport
  Fz : Inport  Port=2
  Mu : Inport  Port=3
  Kt : Inport  Port=4
  Abs : Abs  SaturateOnIntegerOverflow=on
  MuY Front Wheels : Fcn  Expr=(1 - exp(-u(2)*u(1)))
  Mux1 : Mux  Inputs=2
  Product : Product  Inputs=4  SaturateOnIntegerOverflow=on  RndMeth=Zero  InputSameDT=on  OutDataTypeStr=Inherit: Same as first input
  Saturation2 : Saturate  UpperLimit=inf  LowerLimit=1e-9
  Sign : Signum
  Fy : Outport
  wires:
  Abs/1 -> Saturation2/1
  Saturation2/1 -> Mux1/1
  Mux1/1 -> MuY Front Wheels/1
  Kt/1 -> Mux1/2
  Sign/1 -> Product/1
  MuY Front Wheels/1 -> Product/2
  alpha/1 -> Abs/1, Sign/1
  Product/1 -> Fy/1
  Fz/1 -> Product/3
  Mu/1 -> Product/4

== system Demo_CooperativeDriving_cs/Toyota_Yaris_1/Swarm Behavior/Vehicle Dynamics/tyre_forces/tyre_rear/Borstel ==
  alpha : Inport
  Fz : Inport  Port=2
  Mu : Inport  Port=3
  Kt : Inport  Port=4
  Abs : Abs  SaturateOnIntegerOverflow=on
  F : Fcn  Expr=(3*u(2) - 3*u(2)^2 + u(2)^3)*u(1)
  Fmax : Fcn  Expr=u(1)
  Gain : Gain  Gain=1/3  SaturateOnIntegerOverflow=on  OutDataTypeStr=Inherit: Same as input  ParamDataTypeStr=Inherit: Same as input
  Math Function : Math  Operator=reciprocal  SaturateOnIntegerOverflow=on
  Mux1 : Mux  Inputs=2
  Product : Product  SaturateOnIntegerOverflow=on  RndMeth=Zero  InputSameDT=on  OutDataTypeStr=Inherit: Same as first input
  Product1 : Product  Inputs=3  SaturateOnIntegerOverflow=on  RndMeth=Zero  InputSameDT=on  OutDataTypeStr=Inherit: Same as first input
  Relational Operator : RelationalOperator  InputSameDT=on
  Sign : Signum
  Switch : Switch  Threshold=0.5  SaturateOnIntegerOverflow=on  InputSameDT=on
  Trigonometric Function : Trigonometry  Operator=tan
  Fy : Outport
  wires:
  Abs/1 -> Relational Operator/1, Product/1
  Kt/1 -> Gain/1
  Relational Operator/1 -> Switch/2
  Trigonometric Function/1 -> Abs/1
  Mux1/1 -> F/1, Fmax/1
  Sign/1 -> Mux1/1
  Product/1 -> Mux1/2
  F/1 -> Switch/3
  Fmax/1 -> Switch/1
  alpha/1 -> Trigonometric Function/1, Sign/1
  Switch/1 -> Product1/1
  Product1/1 -> Fy/1
  Fz/1 -> Product1/2
  Mu/1 -> Product1/3
  Gain/1 -> Product/2, Math Function/1
  Math Function/1 -> Relational Operator/2

== system Demo_CooperativeDriving_cs/Toyota_Yaris_1/Swarm Behavior/Vehicle Dynamics/tyre_forces/tyre_rear/Exponent ==
  alpha : Inport
  Fz : Inport  Port=2
  Mu : Inport  Port=3
  Kt : Inport  Port=4
  Abs : Abs  SaturateOnIntegerOverflow=on
  MuY Front Wheels : Fcn  Expr=(1 - exp(-u(2)*u(1)))
  Mux1 : Mux  Inputs=2
  Product : Product  Inputs=4  SaturateOnIntegerOverflow=on  RndMeth=Zero  InputSameDT=on  OutDataTypeStr=Inherit: Same as first input
  Saturation2 : Saturate  UpperLimit=inf  LowerLimit=1e-9
  Sign : Signum
  Fy : Outport
  wires:
  Abs/1 -> Saturation2/1
  Saturation2/1 -> Mux1/1
  Mux1/1 -> MuY Front Wheels/1
  Kt/1 -> Mux1/2
  Sign/1 -> Product/1
  MuY Front Wheels/1 -> Product/2
  alpha/1 -> Abs/1, Sign/1
  Product/1 -> Fy/1
  Fz/1 -> Product/3
  Mu/1 -> Product/4
